simulink model "pet_functional_architecture"  (R2024a)
settings: Solver=FixedStepDiscrete  StartTime=0.0  StopTime=10.0  RelTol=1e-3
undefined symbols (not defined in the file): D1, P
(part 2 of 2)

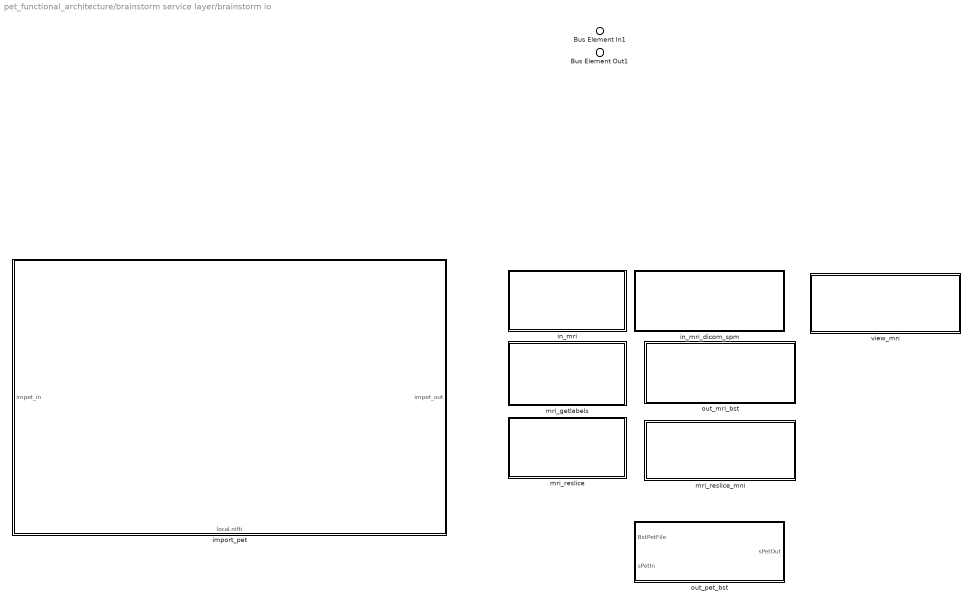
== system pet_functional_architecture/brainstorm service layer/brainstorm io ==
  Bus Element In1 : Inport  AllowServiceAccess=on  PortName=in_(@varargin)
  " out_pet_bst" : Subsystem
      settings: PortSchema="{\"entries\":[{\"content\":{\"headerSize\":26,\"margin\":15,\"minimumSpacing\":25,\"sides\":[{\"content\":{\"connectorIds\":[\"In1\",\"In2\"]},\"type\":\"ConnectorPlacement.EquallySpacedRectSide\",\"uuid\":\"231a4a51-e9d6-4ee1-a9d5-4e29b655c305\"},{\"content\":{\"connectorIds\":[\"Out1\"],\"side\":\"RIGHT\"},\"type\":\"ConnectorPlacement.EquallySpacedRectSide\",\"uuid\":\"e9ceff5f-0784-495f-ae83-524709d043d6\"},{\"content\":{\"side\":\"TOP\"},\"type\":\"ConnectorPlacement.EquallySpacedRectSide\",\"uuid\":\"01c193fb-23d5-46fa-9f50-f56eecaefc77\"}]},\"type\":\"ConnectorPlacement.EquallySpacedConnector\",\"uuid\":\"bc597724-759a-481a-a480-4165a84a707f\"}],\"packageUris\":[\"http://schema.mathworks.com/mf0/Connector/R2020b\"],\"version\":\"1.0\"}"
  import_pet : Subsystem
      settings: PortSchema="{\"entries\":[{\"content\":{\"headerSize\":26,\"margin\":15,\"minimumSpacing\":25,\"sides\":[{\"content\":{\"connectorIds\":[\"In1\"]},\"type\":\"ConnectorPlacement.EquallySpacedRectSide\",\"uuid\":\"e452b68a-48a0-46a4-9e6b-6a7ab63d76ba\"},{\"content\":{\"connectorIds\":[\"Out1\"],\"side\":\"RIGHT\"},\"type\":\"ConnectorPlacement.EquallySpacedRectSide\",\"uuid\":\"bfc23a96-7562-4108-a377-c6d682106293\"},{\"content\":{\"side\":\"TOP\"},\"type\":\"ConnectorPlacement.EquallySpacedRectSide\",\"uuid\":\"898805eb-9365-4e37-9830-3cdbb7191da7\"},{\"content\":{\"connectorIds\":[\"In2\"],\"side\":\"BOTTOM\"},\"type\":\"ConnectorPlacement.EquallySpacedRectSide\",\"uuid\":\"20ed5406-47d9-41fc-b360-c996f9e858c0\"}]},\"type\":\"ConnectorPlacement.EquallySpacedConnector\",\"uuid\":\"9a83eb3e-c81f-4df4-a7ca-e8a116b52f55\"}],\"packageUris\":[\"http://schema.mathworks.com/mf0/Connector/R2020b\"],\"version\":\"1.0\"}"
  in_mri : Subsystem
      settings: PortSchema="{\"entries\":[{\"content\":{\"headerSize\":26,\"margin\":15,\"minimumSpacing\":25,\"sides\":[{\"content\":{},\"type\":\"ConnectorPlacement.EquallySpacedRectSide\",\"uuid\":\"231a4a51-e9d6-4ee1-a9d5-4e29b655c305\"},{\"content\":{\"side\":\"RIGHT\"},\"type\":\"ConnectorPlacement.EquallySpacedRectSide\",\"uuid\":\"e9ceff5f-0784-495f-ae83-524709d043d6\"},{\"content\":{\"side\":\"TOP\"},\"type\":\"ConnectorPlacement.EquallySpacedRectSide\",\"uuid\":\"01c193fb-23d5-46fa-9f50-f56eecaefc77\"}]},\"type\":\"ConnectorPlacement.EquallySpacedConnector\",\"uuid\":\"bc597724-759a-481a-a480-4165a84a707f\"}],\"packageUris\":[\"http://schema.mathworks.com/mf0/Connector/R2020b\"],\"version\":\"1.0\"}"
  in_mri_dicom_spm : Subsystem
      settings: PortSchema="{\"entries\":[{\"content\":{\"headerSize\":26,\"margin\":15,\"minimumSpacing\":25,\"sides\":[{\"content\":{},\"type\":\"ConnectorPlacement.EquallySpacedRectSide\",\"uuid\":\"231a4a51-e9d6-4ee1-a9d5-4e29b655c305\"},{\"content\":{\"side\":\"RIGHT\"},\"type\":\"ConnectorPlacement.EquallySpacedRectSide\",\"uuid\":\"e9ceff5f-0784-495f-ae83-524709d043d6\"},{\"content\":{\"side\":\"TOP\"},\"type\":\"ConnectorPlacement.EquallySpacedRectSide\",\"uuid\":\"01c193fb-23d5-46fa-9f50-f56eecaefc77\"}]},\"type\":\"ConnectorPlacement.EquallySpacedConnector\",\"uuid\":\"bc597724-759a-481a-a480-4165a84a707f\"}],\"packageUris\":[\"http://schema.mathworks.com/mf0/Connector/R2020b\"],\"version\":\"1.0\"}"
  mri_getlabels : Subsystem
      settings: PortSchema="{\"entries\":[{\"content\":{\"headerSize\":26,\"margin\":15,\"minimumSpacing\":25,\"sides\":[{\"content\":{},\"type\":\"ConnectorPlacement.EquallySpacedRectSide\",\"uuid\":\"231a4a51-e9d6-4ee1-a9d5-4e29b655c305\"},{\"content\":{\"side\":\"RIGHT\"},\"type\":\"ConnectorPlacement.EquallySpacedRectSide\",\"uuid\":\"e9ceff5f-0784-495f-ae83-524709d043d6\"},{\"content\":{\"side\":\"TOP\"},\"type\":\"ConnectorPlacement.EquallySpacedRectSide\",\"uuid\":\"01c193fb-23d5-46fa-9f50-f56eecaefc77\"}]},\"type\":\"ConnectorPlacement.EquallySpacedConnector\",\"uuid\":\"bc597724-759a-481a-a480-4165a84a707f\"}],\"packageUris\":[\"http://schema.mathworks.com/mf0/Connector/R2020b\"],\"version\":\"1.0\"}"
  mri_reslice : Subsystem
      settings: PortSchema="{\"entries\":[{\"content\":{\"headerSize\":26,\"margin\":15,\"minimumSpacing\":25,\"sides\":[{\"content\":{},\"type\":\"ConnectorPlacement.EquallySpacedRectSide\",\"uuid\":\"231a4a51-e9d6-4ee1-a9d5-4e29b655c305\"},{\"content\":{\"side\":\"RIGHT\"},\"type\":\"ConnectorPlacement.EquallySpacedRectSide\",\"uuid\":\"e9ceff5f-0784-495f-ae83-524709d043d6\"},{\"content\":{\"side\":\"TOP\"},\"type\":\"ConnectorPlacement.EquallySpacedRectSide\",\"uuid\":\"01c193fb-23d5-46fa-9f50-f56eecaefc77\"}]},\"type\":\"ConnectorPlacement.EquallySpacedConnector\",\"uuid\":\"bc597724-759a-481a-a480-4165a84a707f\"}],\"packageUris\":[\"http://schema.mathworks.com/mf0/Connector/R2020b\"],\"version\":\"1.0\"}"
  mri_reslice_mni : Subsystem
      settings: PortSchema="{\"entries\":[{\"content\":{\"headerSize\":26,\"margin\":15,\"minimumSpacing\":25,\"sides\":[{\"content\":{},\"type\":\"ConnectorPlacement.EquallySpacedRectSide\",\"uuid\":\"231a4a51-e9d6-4ee1-a9d5-4e29b655c305\"},{\"content\":{\"side\":\"RIGHT\"},\"type\":\"ConnectorPlacement.EquallySpacedRectSide\",\"uuid\":\"e9ceff5f-0784-495f-ae83-524709d043d6\"},{\"content\":{\"side\":\"TOP\"},\"type\":\"ConnectorPlacement.EquallySpacedRectSide\",\"uuid\":\"01c193fb-23d5-46fa-9f50-f56eecaefc77\"}]},\"type\":\"ConnectorPlacement.EquallySpacedConnector\",\"uuid\":\"bc597724-759a-481a-a480-4165a84a707f\"}],\"packageUris\":[\"http://schema.mathworks.com/mf0/Connector/R2020b\"],\"version\":\"1.0\"}"
  out_mri_bst : Subsystem
      settings: PortSchema="{\"entries\":[{\"content\":{\"headerSize\":26,\"margin\":15,\"minimumSpacing\":25,\"sides\":[{\"content\":{},\"type\":\"ConnectorPlacement.EquallySpacedRectSide\",\"uuid\":\"231a4a51-e9d6-4ee1-a9d5-4e29b655c305\"},{\"content\":{\"side\":\"RIGHT\"},\"type\":\"ConnectorPlacement.EquallySpacedRectSide\",\"uuid\":\"e9ceff5f-0784-495f-ae83-524709d043d6\"},{\"content\":{\"side\":\"TOP\"},\"type\":\"ConnectorPlacement.EquallySpacedRectSide\",\"uuid\":\"01c193fb-23d5-46fa-9f50-f56eecaefc77\"}]},\"type\":\"ConnectorPlacement.EquallySpacedConnector\",\"uuid\":\"bc597724-759a-481a-a480-4165a84a707f\"}],\"packageUris\":[\"http://schema.mathworks.com/mf0/Connector/R2020b\"],\"version\":\"1.0\"}"
  view_mri : Subsystem
      settings: PortSchema="{\"entries\":[{\"content\":{\"headerSize\":26,\"margin\":15,\"minimumSpacing\":25,\"sides\":[{\"content\":{},\"type\":\"ConnectorPlacement.EquallySpacedRectSide\",\"uuid\":\"231a4a51-e9d6-4ee1-a9d5-4e29b655c305\"},{\"content\":{\"side\":\"RIGHT\"},\"type\":\"ConnectorPlacement.EquallySpacedRectSide\",\"uuid\":\"e9ceff5f-0784-495f-ae83-524709d043d6\"},{\"content\":{\"side\":\"TOP\"},\"type\":\"ConnectorPlacement.EquallySpacedRectSide\",\"uuid\":\"01c193fb-23d5-46fa-9f50-f56eecaefc77\"}]},\"type\":\"ConnectorPlacement.EquallySpacedConnector\",\"uuid\":\"bc597724-759a-481a-a480-4165a84a707f\"}],\"packageUris\":[\"http://schema.mathworks.com/mf0/Connector/R2020b\"],\"version\":\"1.0\"}"
  Bus Element Out1 : Outport  PortName=out_(@varargin)

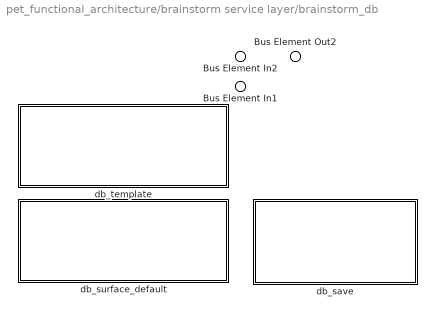
== system pet_functional_architecture/brainstorm service layer/brainstorm_db ==
  Bus Element In1 : Inport  PortName=db_get
  Bus Element In2 : Inport  Port=2  PortName=fcnCall
  db_save : Subsystem
      settings: PortSchema="{\"entries\":[{\"content\":{\"headerSize\":26,\"margin\":15,\"minimumSpacing\":25,\"sides\":[{\"content\":{},\"type\":\"ConnectorPlacement.EquallySpacedRectSide\",\"uuid\":\"231a4a51-e9d6-4ee1-a9d5-4e29b655c305\"},{\"content\":{\"side\":\"RIGHT\"},\"type\":\"ConnectorPlacement.EquallySpacedRectSide\",\"uuid\":\"e9ceff5f-0784-495f-ae83-524709d043d6\"},{\"content\":{\"side\":\"TOP\"},\"type\":\"ConnectorPlacement.EquallySpacedRectSide\",\"uuid\":\"01c193fb-23d5-46fa-9f50-f56eecaefc77\"}]},\"type\":\"ConnectorPlacement.EquallySpacedConnector\",\"uuid\":\"bc597724-759a-481a-a480-4165a84a707f\"}],\"packageUris\":[\"http://schema.mathworks.com/mf0/Connector/R2020b\"],\"version\":\"1.0\"}"
  db_surface_default : Subsystem
      settings: PortSchema="{\"entries\":[{\"content\":{\"headerSize\":26,\"margin\":15,\"minimumSpacing\":25,\"sides\":[{\"content\":{},\"type\":\"ConnectorPlacement.EquallySpacedRectSide\",\"uuid\":\"231a4a51-e9d6-4ee1-a9d5-4e29b655c305\"},{\"content\":{\"side\":\"RIGHT\"},\"type\":\"ConnectorPlacement.EquallySpacedRectSide\",\"uuid\":\"e9ceff5f-0784-495f-ae83-524709d043d6\"},{\"content\":{\"side\":\"TOP\"},\"type\":\"ConnectorPlacement.EquallySpacedRectSide\",\"uuid\":\"01c193fb-23d5-46fa-9f50-f56eecaefc77\"}]},\"type\":\"ConnectorPlacement.EquallySpacedConnector\",\"uuid\":\"bc597724-759a-481a-a480-4165a84a707f\"}],\"packageUris\":[\"http://schema.mathworks.com/mf0/Connector/R2020b\"],\"version\":\"1.0\"}"
  db_template : Subsystem
      settings: PortSchema="{\"entries\":[{\"content\":{\"headerSize\":26,\"margin\":15,\"minimumSpacing\":25,\"sides\":[{\"content\":{},\"type\":\"ConnectorPlacement.EquallySpacedRectSide\",\"uuid\":\"231a4a51-e9d6-4ee1-a9d5-4e29b655c305\"},{\"content\":{\"side\":\"RIGHT\"},\"type\":\"ConnectorPlacement.EquallySpacedRectSide\",\"uuid\":\"e9ceff5f-0784-495f-ae83-524709d043d6\"},{\"content\":{\"side\":\"TOP\"},\"type\":\"ConnectorPlacement.EquallySpacedRectSide\",\"uuid\":\"01c193fb-23d5-46fa-9f50-f56eecaefc77\"}]},\"type\":\"ConnectorPlacement.EquallySpacedConnector\",\"uuid\":\"bc597724-759a-481a-a480-4165a84a707f\"}],\"packageUris\":[\"http://schema.mathworks.com/mf0/Connector/R2020b\"],\"version\":\"1.0\"}"
  Bus Element Out2 : Outport  PortName=db_set

== system pet_functional_architecture/brainstorm tools/ java_getfile ==

== system pet_functional_architecture/brainstorm tools/Anatomy ==
  Bus Element Out2 : Outport  AllowServiceAccess=on  PortName=Surface Recon
  Bus Element Out1 : Outport  Port=2  AllowServiceAccess=on  PortName=BstMriFile

== system pet_functional_architecture/brainstorm tools/bst_colormaps ==

== system pet_functional_architecture/brainstorm tools/bst_fileparts ==

== system pet_functional_architecture/brainstorm tools/bst_flip ==

== system pet_functional_architecture/brainstorm tools/bst_fullfile ==

== system pet_functional_architecture/brainstorm tools/bst_get ==
  Bus Element In2 : Inport  PortName=bst_get(@db)
  Out Bus Element1 : Outport  PortName=io

== system pet_functional_architecture/brainstorm tools/bst_history ==

== system pet_functional_architecture/brainstorm tools/bst_memory ==

== system pet_functional_architecture/brainstorm tools/bst_progress ==

== system pet_functional_architecture/brainstorm tools/bst_set ==
  Bus Element In1 : Inport  PortName=io
  Out Bus Element1 : Outport  PortName=bst_set(@db)

== system pet_functional_architecture/brainstorm tools/db_save ==

== system pet_functional_architecture/brainstorm tools/db_surface_default ==

== system pet_functional_architecture/brainstorm tools/db_template ==

== system pet_functional_architecture/brainstorm tools/file_delete ==

== system pet_functional_architecture/brainstorm tools/file_expand_selection ==

== system pet_functional_architecture/brainstorm tools/file_standardize ==

== system pet_functional_architecture/brainstorm tools/in_mri ==

== system pet_functional_architecture/brainstorm tools/in_mri_dicom_spm ==

== system pet_functional_architecture/brainstorm tools/java_dialog ==

== system pet_functional_architecture/brainstorm tools/mri_getlabels ==

== system pet_functional_architecture/brainstorm tools/mri_reslice ==

== system pet_functional_architecture/brainstorm tools/mri_reslice_mni ==

== system pet_functional_architecture/brainstorm tools/out_mri_bst ==

== system pet_functional_architecture/brainstorm tools/panel_protocols ==

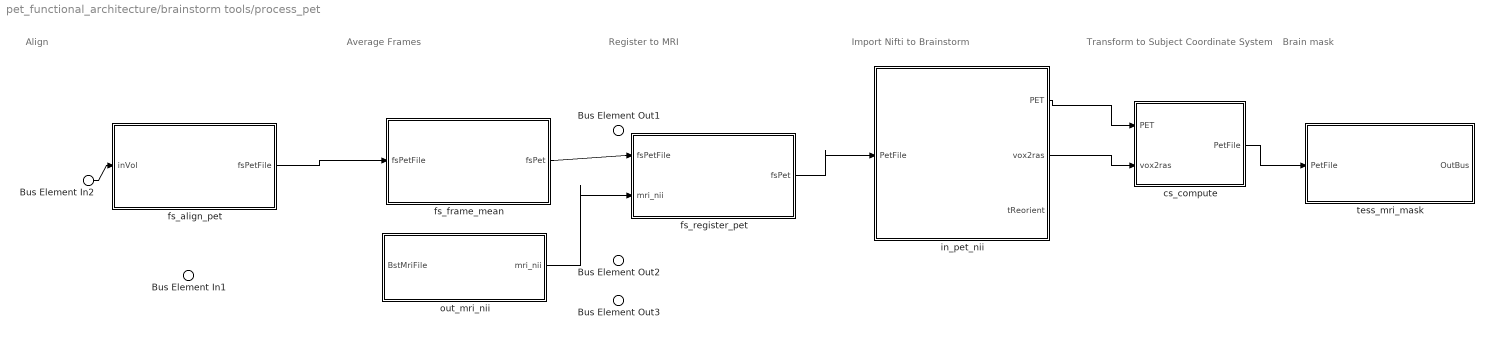
== system pet_functional_architecture/brainstorm tools/process_pet ==
  note: Average Frames
  note: Import Nifti to Brainstorm
  note: Brain mask
  note: Register to MRI
  note: Align
  note: Transform to
      | Subject Coordinate System
  Bus Element In2 : Inport  PortName=PetFile
  Bus Element In1 : Inport  Port=2  AllowServiceAccess=on  PortName=BstMriFile
  cs_compute : Subsystem
      settings: PortSchema="{\"entries\":[{\"content\":{\"headerSize\":26,\"margin\":15,\"minimumSpacing\":25,\"sides\":[{\"content\":{\"connectorIds\":[\"In1\",\"In2\"]},\"type\":\"ConnectorPlacement.EquallySpacedRectSide\",\"uuid\":\"d9face5b-155e-4e83-95c0-d581b737b6e3\"},{\"content\":{\"connectorIds\":[\"Out1\"],\"side\":\"RIGHT\"},\"type\":\"ConnectorPlacement.EquallySpacedRectSide\",\"uuid\":\"f965be1f-1639-4140-b9ea-f5e9efbe4150\"},{\"content\":{\"side\":\"TOP\"},\"type\":\"ConnectorPlacement.EquallySpacedRectSide\",\"uuid\":\"7c9c4b2b-011c-4482-afab-b6e67025a5e2\"}]},\"type\":\"ConnectorPlacement.EquallySpacedConnector\",\"uuid\":\"ec963004-117d-4f22-bb00-71f35201e6e2\"}],\"packageUris\":[\"http://schema.mathworks.com/mf0/Connector/R2020b\"],\"version\":\"1.0\"}"
  fs_align_pet : Subsystem
      settings: PortSchema="{\"entries\":[{\"content\":{\"headerSize\":26,\"margin\":15,\"minimumSpacing\":25,\"sides\":[{\"content\":{\"connectorIds\":[\"In1\"]},\"type\":\"ConnectorPlacement.EquallySpacedRectSide\",\"uuid\":\"d9face5b-155e-4e83-95c0-d581b737b6e3\"},{\"content\":{\"connectorIds\":[\"Out1\"],\"side\":\"RIGHT\"},\"type\":\"ConnectorPlacement.EquallySpacedRectSide\",\"uuid\":\"f965be1f-1639-4140-b9ea-f5e9efbe4150\"},{\"content\":{\"side\":\"TOP\"},\"type\":\"ConnectorPlacement.EquallySpacedRectSide\",\"uuid\":\"7c9c4b2b-011c-4482-afab-b6e67025a5e2\"}]},\"type\":\"ConnectorPlacement.EquallySpacedConnector\",\"uuid\":\"ec963004-117d-4f22-bb00-71f35201e6e2\"}],\"packageUris\":[\"http://schema.mathworks.com/mf0/Connector/R2020b\"],\"version\":\"1.0\"}"
  fs_frame_mean : Subsystem
      settings: PortSchema="{\"entries\":[{\"content\":{\"headerSize\":26,\"margin\":15,\"minimumSpacing\":25,\"sides\":[{\"content\":{\"connectorIds\":[\"In1\"]},\"type\":\"ConnectorPlacement.EquallySpacedRectSide\",\"uuid\":\"d9face5b-155e-4e83-95c0-d581b737b6e3\"},{\"content\":{\"connectorIds\":[\"Out1\"],\"side\":\"RIGHT\"},\"type\":\"ConnectorPlacement.EquallySpacedRectSide\",\"uuid\":\"f965be1f-1639-4140-b9ea-f5e9efbe4150\"},{\"content\":{\"side\":\"TOP\"},\"type\":\"ConnectorPlacement.EquallySpacedRectSide\",\"uuid\":\"7c9c4b2b-011c-4482-afab-b6e67025a5e2\"}]},\"type\":\"ConnectorPlacement.EquallySpacedConnector\",\"uuid\":\"ec963004-117d-4f22-bb00-71f35201e6e2\"}],\"packageUris\":[\"http://schema.mathworks.com/mf0/Connector/R2020b\"],\"version\":\"1.0\"}"
  fs_register_pet : Subsystem
      settings: PortSchema="{\"entries\":[{\"content\":{\"headerSize\":26,\"margin\":15,\"minimumSpacing\":25,\"sides\":[{\"content\":{\"connectorIds\":[\"In1\",\"In2\"]},\"type\":\"ConnectorPlacement.EquallySpacedRectSide\",\"uuid\":\"d9face5b-155e-4e83-95c0-d581b737b6e3\"},{\"content\":{\"connectorIds\":[\"Out1\"],\"side\":\"RIGHT\"},\"type\":\"ConnectorPlacement.EquallySpacedRectSide\",\"uuid\":\"f965be1f-1639-4140-b9ea-f5e9efbe4150\"},{\"content\":{\"side\":\"TOP\"},\"type\":\"ConnectorPlacement.EquallySpacedRectSide\",\"uuid\":\"7c9c4b2b-011c-4482-afab-b6e67025a5e2\"}]},\"type\":\"ConnectorPlacement.EquallySpacedConnector\",\"uuid\":\"ec963004-117d-4f22-bb00-71f35201e6e2\"}],\"packageUris\":[\"http://schema.mathworks.com/mf0/Connector/R2020b\"],\"version\":\"1.0\"}"
  in_pet_nii : Subsystem
      settings: PortSchema="{\"entries\":[{\"content\":{\"headerSize\":26,\"margin\":15,\"minimumSpacing\":25,\"sides\":[{\"content\":{\"connectorIds\":[\"In1\"]},\"type\":\"ConnectorPlacement.EquallySpacedRectSide\",\"uuid\":\"d9face5b-155e-4e83-95c0-d581b737b6e3\"},{\"content\":{\"connectorIds\":[\"Out1\",\"Out2\",\"Out3\"],\"side\":\"RIGHT\"},\"type\":\"ConnectorPlacement.EquallySpacedRectSide\",\"uuid\":\"f965be1f-1639-4140-b9ea-f5e9efbe4150\"},{\"content\":{\"side\":\"TOP\"},\"type\":\"ConnectorPlacement.EquallySpacedRectSide\",\"uuid\":\"7c9c4b2b-011c-4482-afab-b6e67025a5e2\"}]},\"type\":\"ConnectorPlacement.EquallySpacedConnector\",\"uuid\":\"ec963004-117d-4f22-bb00-71f35201e6e2\"}],\"packageUris\":[\"http://schema.mathworks.com/mf0/Connector/R2020b\"],\"version\":\"1.0\"}"
  out_mri_nii : Subsystem
      settings: PortSchema="{\"entries\":[{\"content\":{\"headerSize\":26,\"margin\":15,\"minimumSpacing\":25,\"sides\":[{\"content\":{\"connectorIds\":[\"In1\"]},\"type\":\"ConnectorPlacement.EquallySpacedRectSide\",\"uuid\":\"d9face5b-155e-4e83-95c0-d581b737b6e3\"},{\"content\":{\"connectorIds\":[\"Out1\"],\"side\":\"RIGHT\"},\"type\":\"ConnectorPlacement.EquallySpacedRectSide\",\"uuid\":\"f965be1f-1639-4140-b9ea-f5e9efbe4150\"},{\"content\":{\"side\":\"TOP\"},\"type\":\"ConnectorPlacement.EquallySpacedRectSide\",\"uuid\":\"7c9c4b2b-011c-4482-afab-b6e67025a5e2\"}]},\"type\":\"ConnectorPlacement.EquallySpacedConnector\",\"uuid\":\"ec963004-117d-4f22-bb00-71f35201e6e2\"}],\"packageUris\":[\"http://schema.mathworks.com/mf0/Connector/R2020b\"],\"version\":\"1.0\"}"
  tess_mri_mask : Subsystem
      settings: PortSchema="{\"entries\":[{\"content\":{\"headerSize\":26,\"margin\":15,\"minimumSpacing\":25,\"sides\":[{\"content\":{\"connectorIds\":[\"In1\"]},\"type\":\"ConnectorPlacement.EquallySpacedRectSide\",\"uuid\":\"d9face5b-155e-4e83-95c0-d581b737b6e3\"},{\"content\":{\"connectorIds\":[\"Out1\"],\"side\":\"RIGHT\"},\"type\":\"ConnectorPlacement.EquallySpacedRectSide\",\"uuid\":\"f965be1f-1639-4140-b9ea-f5e9efbe4150\"},{\"content\":{\"side\":\"TOP\"},\"type\":\"ConnectorPlacement.EquallySpacedRectSide\",\"uuid\":\"7c9c4b2b-011c-4482-afab-b6e67025a5e2\"}]},\"type\":\"ConnectorPlacement.EquallySpacedConnector\",\"uuid\":\"ec963004-117d-4f22-bb00-71f35201e6e2\"}],\"packageUris\":[\"http://schema.mathworks.com/mf0/Connector/R2020b\"],\"version\":\"1.0\"}"
  Bus Element Out1 : Outport  PortName=sPet
  Bus Element Out2 : Outport  Port=2  PortName=SUVR Volume
  Bus Element Out3 : Outport  Port=3  PortName=Surface Overlay
  wires:
  Bus Element In2/1 -> fs_align_pet/1(inVol)
  out_mri_nii/1(mri_nii) -> fs_register_pet/2(mri_nii)
  fs_align_pet/1(fsPetFile) -> fs_frame_mean/1(fsPetFile)
  in_pet_nii/2(vox2ras) -> cs_compute/2(vox2ras)
  in_pet_nii/1(PET) -> cs_compute/1(PET)
  fs_frame_mean/1(fsPet) -> fs_register_pet/1(fsPetFile)
  fs_register_pet/1(fsPet) -> in_pet_nii/1(PetFile)
  cs_compute/1(PetFile) -> tess_mri_mask/1(PetFile)

== system pet_functional_architecture/brainstorm tools/view_mri ==

== system pet_functional_architecture/Freesurfer//Brainsuite/Freesurfer/LORIS Data Ingestor ==

== system pet_functional_architecture/Freesurfer//Brainsuite/Freesurfer/Linux ==
  Bus Element In1 : Inport  AllowServiceAccess=on  PortName=Client

== system pet_functional_architecture/Freesurfer//Brainsuite/Freesurfer/Windows ==
  Bus Element In1 : Inport  AllowServiceAccess=on  PortName=Client

== system pet_functional_architecture/Freesurfer//Brainsuite/Freesurfer/gitClone Brainstorm ==
  Bus Element In1 : Inport  AllowServiceAccess=on  PortName=sourceCode

== system pet_functional_architecture/brainstorm service layer/brainstorm core/bst_colormaps ==

== system pet_functional_architecture/brainstorm service layer/brainstorm core/bst_fileparts ==

== system pet_functional_architecture/brainstorm service layer/brainstorm core/bst_flip ==

== system pet_functional_architecture/brainstorm service layer/brainstorm core/bst_fullfile ==

== system pet_functional_architecture/brainstorm service layer/brainstorm core/bst_get ==

== system pet_functional_architecture/brainstorm service layer/brainstorm core/bst_get1 ==
  Bus Element In2 : Inport  PortName=bst_get(@db)
  Out Bus Element1 : Outport  PortName=io

== system pet_functional_architecture/brainstorm service layer/brainstorm core/bst_history ==

== system pet_functional_architecture/brainstorm service layer/brainstorm core/bst_memory ==

== system pet_functional_architecture/brainstorm service layer/brainstorm core/bst_progress ==

== system pet_functional_architecture/brainstorm service layer/brainstorm core/bst_set ==

== system pet_functional_architecture/brainstorm service layer/brainstorm core/bst_set1 ==
  Bus Element In1 : Inport  PortName=io
  Out Bus Element1 : Outport  PortName=bst_set(@db)

== system pet_functional_architecture/brainstorm service layer/brainstorm io/ out_pet_bst ==
  Bus Element In2 : Inport  PortName=BstPetFile
  Bus Element In1 : Inport  Port=2  PortName=sPetIn
  Bus Element Out1 : Outport  PortName=sPetOut

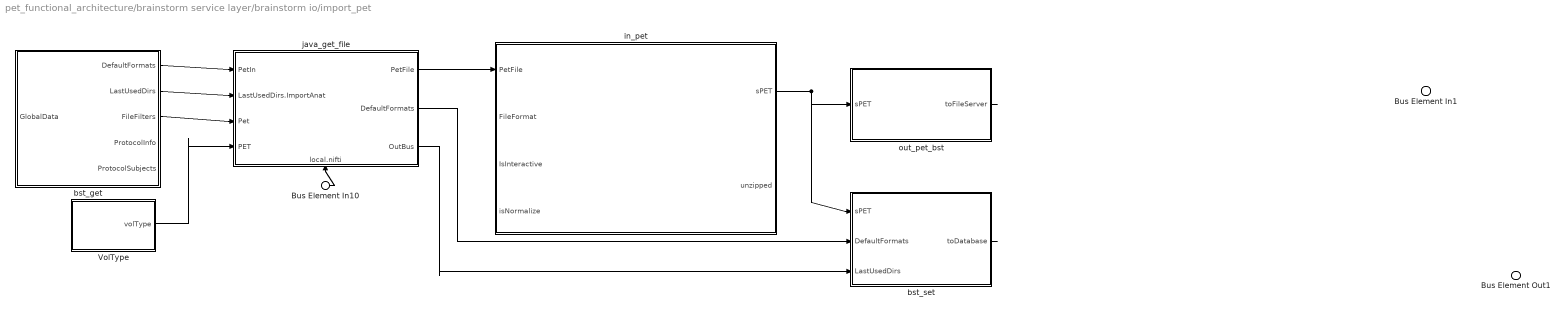
== system pet_functional_architecture/brainstorm service layer/brainstorm io/import_pet ==
  Bus Element In1 : Inport  PortName=impet_in
  Bus Element In10 : Inport  Port=2  AllowServiceAccess=on  PortName=local.nifti
  VolType : Subsystem
      settings: PortSchema="{\"entries\":[{\"content\":{\"headerSize\":26,\"margin\":15,\"minimumSpacing\":25,\"sides\":[{\"content\":{},\"type\":\"ConnectorPlacement.EquallySpacedRectSide\",\"uuid\":\"9dc41937-0423-4f0d-95de-6a11876dea92\"},{\"content\":{\"connectorIds\":[\"Out1\"],\"side\":\"RIGHT\"},\"type\":\"ConnectorPlacement.EquallySpacedRectSide\",\"uuid\":\"a760f902-bb88-44c6-9e15-f93a06bbb22c\"},{\"content\":{\"side\":\"TOP\"},\"type\":\"ConnectorPlacement.EquallySpacedRectSide\",\"uuid\":\"a141426c-a194-4d5c-ba1a-f6f4f49c40a6\"}]},\"type\":\"ConnectorPlacement.EquallySpacedConnector\",\"uuid\":\"ec924d27-401c-47e0-a07a-aece678b254f\"}],\"packageUris\":[\"http://schema.mathworks.com/mf0/Connector/R2020b\"],\"version\":\"1.0\"}"
  bst_get : Subsystem
      settings: PortSchema="{\"entries\":[{\"content\":{\"headerSize\":26,\"margin\":15,\"minimumSpacing\":25,\"sides\":[{\"content\":{\"connectorIds\":[\"In1\"]},\"type\":\"ConnectorPlacement.EquallySpacedRectSide\",\"uuid\":\"e452b68a-48a0-46a4-9e6b-6a7ab63d76ba\"},{\"content\":{\"connectorIds\":[\"Out1\",\"Out2\",\"Out3\",\"Out4\",\"Out5\"],\"side\":\"RIGHT\"},\"type\":\"ConnectorPlacement.EquallySpacedRectSide\",\"uuid\":\"bfc23a96-7562-4108-a377-c6d682106293\"},{\"content\":{\"side\":\"TOP\"},\"type\":\"ConnectorPlacement.EquallySpacedRectSide\",\"uuid\":\"898805eb-9365-4e37-9830-3cdbb7191da7\"}]},\"type\":\"ConnectorPlacement.EquallySpacedConnector\",\"uuid\":\"9a83eb3e-c81f-4df4-a7ca-e8a116b52f55\"}],\"packageUris\":[\"http://schema.mathworks.com/mf0/Connector/R2020b\"],\"version\":\"1.0\"}"
  bst_set : Subsystem
      settings: PortSchema="{\"entries\":[{\"content\":{\"headerSize\":26,\"margin\":15,\"minimumSpacing\":25,\"sides\":[{\"content\":{\"connectorIds\":[\"In1\",\"In2\",\"In3\"]},\"type\":\"ConnectorPlacement.EquallySpacedRectSide\",\"uuid\":\"e452b68a-48a0-46a4-9e6b-6a7ab63d76ba\"},{\"content\":{\"connectorIds\":[\"Out1\"],\"side\":\"RIGHT\"},\"type\":\"ConnectorPlacement.EquallySpacedRectSide\",\"uuid\":\"bfc23a96-7562-4108-a377-c6d682106293\"},{\"content\":{\"side\":\"TOP\"},\"type\":\"ConnectorPlacement.EquallySpacedRectSide\",\"uuid\":\"898805eb-9365-4e37-9830-3cdbb7191da7\"}]},\"type\":\"ConnectorPlacement.EquallySpacedConnector\",\"uuid\":\"9a83eb3e-c81f-4df4-a7ca-e8a116b52f55\"}],\"packageUris\":[\"http://schema.mathworks.com/mf0/Connector/R2020b\"],\"version\":\"1.0\"}"
  in_pet : Subsystem
      settings: PortSchema="{\"entries\":[{\"content\":{\"headerSize\":26,\"margin\":15,\"minimumSpacing\":25,\"sides\":[{\"content\":{\"connectorIds\":[\"In4\",\"In1\",\"In2\",\"In3\"]},\"type\":\"ConnectorPlacement.EquallySpacedRectSide\",\"uuid\":\"e452b68a-48a0-46a4-9e6b-6a7ab63d76ba\"},{\"content\":{\"connectorIds\":[\"Out1\",\"Out2\"],\"side\":\"RIGHT\"},\"type\":\"ConnectorPlacement.EquallySpacedRectSide\",\"uuid\":\"bfc23a96-7562-4108-a377-c6d682106293\"},{\"content\":{\"side\":\"TOP\"},\"type\":\"ConnectorPlacement.EquallySpacedRectSide\",\"uuid\":\"898805eb-9365-4e37-9830-3cdbb7191da7\"}]},\"type\":\"ConnectorPlacement.EquallySpacedConnector\",\"uuid\":\"9a83eb3e-c81f-4df4-a7ca-e8a116b52f55\"}],\"packageUris\":[\"http://schema.mathworks.com/mf0/Connector/R2020b\"],\"version\":\"1.0\"}"
  java_get_file : Subsystem
      settings: PortSchema="{\"entries\":[{\"content\":{\"headerSize\":26,\"margin\":15,\"minimumSpacing\":25,\"sides\":[{\"content\":{\"connectorIds\":[\"In2\",\"In1\",\"In3\",\"In4\"]},\"type\":\"ConnectorPlacement.EquallySpacedRectSide\",\"uuid\":\"d9face5b-155e-4e83-95c0-d581b737b6e3\"},{\"content\":{\"connectorIds\":[\"Out1\",\"Out2\",\"Out3\"],\"side\":\"RIGHT\"},\"type\":\"ConnectorPlacement.EquallySpacedRectSide\",\"uuid\":\"f965be1f-1639-4140-b9ea-f5e9efbe4150\"},{\"content\":{\"side\":\"TOP\"},\"type\":\"ConnectorPlacement.EquallySpacedRectSide\",\"uuid\":\"7c9c4b2b-011c-4482-afab-b6e67025a5e2\"},{\"content\":{\"connectorIds\":[\"In5\"],\"side\":\"BOTTOM\"},\"type\":\"ConnectorPlacement.EquallySpacedRectSide\",\"uuid\":\"d045f323-f36b-4304-ab53-40ed85860a49\"}]},\"type\":\"ConnectorPlacement.EquallySpacedConnector\",\"uuid\":\"ec963004-117d-4f22-bb00-71f35201e6e2\"}],\"packageUris\":[\"http://schema.mathworks.com/mf0/Connector/R2020b\"],\"version\":\"1.0\"}"
  out_pet_bst : Subsystem
      settings: PortSchema="{\"entries\":[{\"content\":{\"headerSize\":26,\"margin\":15,\"minimumSpacing\":25,\"sides\":[{\"content\":{\"connectorIds\":[\"In1\"]},\"type\":\"ConnectorPlacement.EquallySpacedRectSide\",\"uuid\":\"b493315f-c6c8-42ab-8e4d-b8fe240af9dd\"},{\"content\":{\"connectorIds\":[\"Out1\"],\"side\":\"RIGHT\"},\"type\":\"ConnectorPlacement.EquallySpacedRectSide\",\"uuid\":\"94c0e42b-c474-4070-8a16-a26ac22942e6\"},{\"content\":{\"side\":\"TOP\"},\"type\":\"ConnectorPlacement.EquallySpacedRectSide\",\"uuid\":\"f9bc43e9-5c3a-451c-b434-9225c48927cc\"}]},\"type\":\"ConnectorPlacement.EquallySpacedConnector\",\"uuid\":\"067458af-ee7c-44e6-8802-98d558b25815\"}],\"packageUris\":[\"http://schema.mathworks.com/mf0/Connector/R2020b\"],\"version\":\"1.0\"}"
  Bus Element Out1 : Outport  PortName=impet_out
  wires:
  bst_get/3(FileFilters) -> java_get_file/3(Pet)
  bst_get/2(LastUsedDirs) -> java_get_file/1(LastUsedDirs.ImportAnat)
  bst_get/1(DefaultFormats) -> java_get_file/2(PetIn)
  Bus Element In10/1 -> java_get_file/5(local.nifti)
  java_get_file/1(PetFile) -> in_pet/4(PetFile)
  java_get_file/2(DefaultFormats) -> bst_set/2(DefaultFormats)
  java_get_file/3(OutBus) -> bst_set/3(LastUsedDirs)
  VolType/1(volType) -> java_get_file/4(PET)
  in_pet/1(sPET) -> bst_set/1(sPET), out_pet_bst/1(sPET)
  out_pet_bst/1(toFileServer) -> ?
  bst_set/1(toDatabase) -> ?

== system pet_functional_architecture/brainstorm service layer/brainstorm io/in_mri ==

== system pet_functional_architecture/brainstorm service layer/brainstorm io/in_mri_dicom_spm ==

== system pet_functional_architecture/brainstorm service layer/brainstorm io/mri_getlabels ==

== system pet_functional_architecture/brainstorm service layer/brainstorm io/mri_reslice ==

== system pet_functional_architecture/brainstorm service layer/brainstorm io/mri_reslice_mni ==

== system pet_functional_architecture/brainstorm service layer/brainstorm io/out_mri_bst ==

== system pet_functional_architecture/brainstorm service layer/brainstorm io/view_mri ==

== system pet_functional_architecture/brainstorm service layer/brainstorm_db/db_save ==

== system pet_functional_architecture/brainstorm service layer/brainstorm_db/db_surface_default ==

== system pet_functional_architecture/brainstorm service layer/brainstorm_db/db_template ==

== system pet_functional_architecture/brainstorm tools/process_pet/cs_compute ==
  Bus Element In1 : Inport  PortName=PET
  Bus Element In2 : Inport  Port=2  PortName=vox2ras
  Bus Element Out1 : Outport  PortName=PetFile

== system pet_functional_architecture/brainstorm tools/process_pet/fs_align_pet ==
  Bus Element In1 : Inport  PortName=inVol
  Bus Element Out1 : Outport  PortName=fsPetFile

== system pet_functional_architecture/brainstorm tools/process_pet/fs_frame_mean ==
  Bus Element In1 : Inport  PortName=fsPetFile
  Bus Element Out1 : Outport  PortName=fsPet

== system pet_functional_architecture/brainstorm tools/process_pet/fs_register_pet ==
  Bus Element In1 : Inport  PortName=fsPetFile
  Bus Element In2 : Inport  Port=2  PortName=mri_nii
  Bus Element Out1 : Outport  PortName=fsPet

== system pet_functional_architecture/brainstorm tools/process_pet/in_pet_nii ==
  Bus Element In1 : Inport  PortName=PetFile
  Bus Element Out1 : Outport  PortName=PET
  Bus Element Out2 : Outport  Port=2  PortName=vox2ras
  Bus Element Out3 : Outport  Port=3  PortName=tReorient

== system pet_functional_architecture/brainstorm tools/process_pet/out_mri_nii ==
  Bus Element In1 : Inport  AllowServiceAccess=on  PortName=BstMriFile
  Bus Element Out1 : Outport  PortName=mri_nii

== system pet_functional_architecture/brainstorm tools/process_pet/tess_mri_mask ==
  Bus Element In1 : Inport  PortName=PetFile
  Bus Element Out1 : Outport  PortName=OutBus

== system pet_functional_architecture/brainstorm service layer/brainstorm io/import_pet/VolType ==
  Bus Element Out1 : Outport  PortName=volType

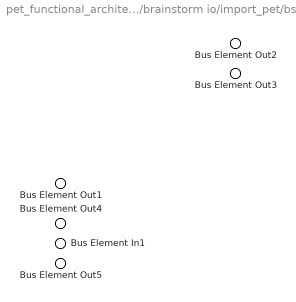
== system pet_functional_architecture/brainstorm service layer/brainstorm io/import_pet/bst_get ==
  Bus Element In1 : Inport  PortName=GlobalData
  Bus Element Out3 : Outport  PortName=DefaultFormats
  Bus Element Out2 : Outport  Port=2  PortName=LastUsedDirs
  Bus Element Out1 : Outport  Port=3  PortName=FileFilters
  Bus Element Out4 : Outport  Port=4  PortName=ProtocolInfo
  Bus Element Out5 : Outport  Port=5  PortName=ProtocolSubjects

== system pet_functional_architecture/brainstorm service layer/brainstorm io/import_pet/bst_set ==
  Bus Element In3 : Inport  PortName=sPET
  Bus Element In1 : Inport  Port=2  PortName=DefaultFormats
  Bus Element In2 : Inport  Port=3  PortName=LastUsedDirs
  Bus Element Out1 : Outport  PortName=toDatabase

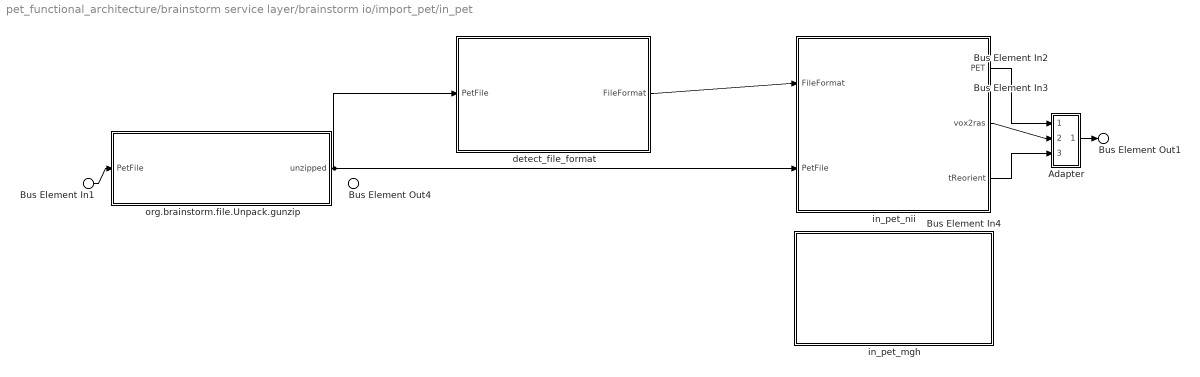
== system pet_functional_architecture/brainstorm service layer/brainstorm io/import_pet/in_pet ==
  Bus Element In2 : Inport  PortName=FileFormat
  Bus Element In3 : Inport  Port=2  PortName=IsInteractive
  Bus Element In4 : Inport  Port=3  PortName=isNormalize
  Bus Element In1 : Inport  Port=4  PortName=PetFile
  Adapter : Subsystem
      settings: PortSchema="{\"entries\":[{\"content\":{\"margin\":10,\"minimumSpacing\":15,\"sides\":[{\"content\":{\"connectorIds\":[\"In1\",\"In2\",\"In3\"]},\"type\":\"ConnectorPlacement.EquallySpacedRectSide\",\"uuid\":\"b493315f-c6c8-42ab-8e4d-b8fe240af9dd\"},{\"content\":{\"connectorIds\":[\"Out1\"],\"side\":\"RIGHT\"},\"type\":\"ConnectorPlacement.EquallySpacedRectSide\",\"uuid\":\"94c0e42b-c474-4070-8a16-a26ac22942e6\"},{\"content\":{\"side\":\"TOP\"},\"type\":\"ConnectorPlacement.EquallySpacedRectSide\",\"uuid\":\"f9bc43e9-5c3a-451c-b434-9225c48927cc\"}]},\"type\":\"ConnectorPlacement.EquallySpacedConnector\",\"uuid\":\"067458af-ee7c-44e6-8802-98d558b25815\"}],\"packageUris\":[\"http://schema.mathworks.com/mf0/Connector/R2020b\"],\"version\":\"1.0\"}"
  detect_file_format : Subsystem
      settings: AttributesFormatString=%<BlockChoice>  PortSchema="{\"entries\":[{\"content\":{\"headerSize\":26,\"margin\":15,\"minimumSpacing\":25,\"sides\":[{\"content\":{\"connectorIds\":[\"In1\"]},\"type\":\"ConnectorPlacement.EquallySpacedRectSide\",\"uuid\":\"e452b68a-48a0-46a4-9e6b-6a7ab63d76ba\"},{\"content\":{\"connectorIds\":[\"Out1\"],\"side\":\"RIGHT\"},\"type\":\"ConnectorPlacement.EquallySpacedRectSide\",\"uuid\":\"bfc23a96-7562-4108-a377-c6d682106293\"},{\"content\":{\"side\":\"TOP\"},\"type\":\"ConnectorPlacement.EquallySpacedRectSide\",\"uuid\":\"898805eb-9365-4e37-9830-3cdbb7191da7\"}]},\"type\":\"ConnectorPlacement.EquallySpacedConnector\",\"uuid\":\"9a83eb3e-c81f-4df4-a7ca-e8a116b52f55\"}],\"packageUris\":[\"http://schema.mathworks.com/mf0/Connector/R2020b\"],\"version\":\"1.0\"}"
  in_pet_mgh : Subsystem  Variant=on  VariantControlMode=label  LabelModeActiveChoice=true
      settings: PortSchema="{\"entries\":[{\"content\":{\"headerSize\":38,\"margin\":15,\"minimumSpacing\":25,\"sides\":[{\"content\":{},\"type\":\"ConnectorPlacement.EquallySpacedRectSide\",\"uuid\":\"b5ae5544-e8bb-4254-ad00-58833e8a7a18\"},{\"content\":{\"side\":\"RIGHT\"},\"type\":\"ConnectorPlacement.EquallySpacedRectSide\",\"uuid\":\"fac4f2c4-a4bc-47a5-a441-dcd98ce2bd10\"},{\"content\":{\"side\":\"TOP\"},\"type\":\"ConnectorPlacement.EquallySpacedRectSide\",\"uuid\":\"59b20440-0331-47da-a238-f55a29059bc4\"}]},\"type\":\"ConnectorPlacement.EquallySpacedConnector\",\"uuid\":\"540bd42e-d22d-4480-8642-7df807d4afe7\"}],\"packageUris\":[\"http://schema.mathworks.com/mf0/Connector/R2020b\"],\"version\":\"1.0\"}"
  in_pet_nii : Subsystem
      settings: PortSchema="{\"entries\":[{\"content\":{\"headerSize\":26,\"margin\":15,\"minimumSpacing\":25,\"sides\":[{\"content\":{\"connectorIds\":[\"In1\",\"In2\"]},\"type\":\"ConnectorPlacement.EquallySpacedRectSide\",\"uuid\":\"9dc41937-0423-4f0d-95de-6a11876dea92\"},{\"content\":{\"connectorIds\":[\"Out1\",\"Out2\",\"Out3\"],\"side\":\"RIGHT\"},\"type\":\"ConnectorPlacement.EquallySpacedRectSide\",\"uuid\":\"a760f902-bb88-44c6-9e15-f93a06bbb22c\"},{\"content\":{\"side\":\"TOP\"},\"type\":\"ConnectorPlacement.EquallySpacedRectSide\",\"uuid\":\"a141426c-a194-4d5c-ba1a-f6f4f49c40a6\"}]},\"type\":\"ConnectorPlacement.EquallySpacedConnector\",\"uuid\":\"ec924d27-401c-47e0-a07a-aece678b254f\"}],\"packageUris\":[\"http://schema.mathworks.com/mf0/Connector/R2020b\"],\"version\":\"1.0\"}"
  org.brainstorm.file.Unpack.gunzip : Subsystem
      settings: PortSchema="{\"entries\":[{\"content\":{\"headerSize\":26,\"margin\":15,\"minimumSpacing\":25,\"sides\":[{\"content\":{\"connectorIds\":[\"In1\"]},\"type\":\"ConnectorPlacement.EquallySpacedRectSide\",\"uuid\":\"e452b68a-48a0-46a4-9e6b-6a7ab63d76ba\"},{\"content\":{\"connectorIds\":[\"Out1\"],\"side\":\"RIGHT\"},\"type\":\"ConnectorPlacement.EquallySpacedRectSide\",\"uuid\":\"bfc23a96-7562-4108-a377-c6d682106293\"},{\"content\":{\"side\":\"TOP\"},\"type\":\"ConnectorPlacement.EquallySpacedRectSide\",\"uuid\":\"898805eb-9365-4e37-9830-3cdbb7191da7\"},{\"content\":{\"side\":\"BOTTOM\"},\"type\":\"ConnectorPlacement.EquallySpacedRectSide\",\"uuid\":\"c4b35227-9c6e-45b4-8456-8559ba2769ae\"}]},\"type\":\"ConnectorPlacement.EquallySpacedConnector\",\"uuid\":\"9a83eb3e-c81f-4df4-a7ca-e8a116b52f55\"}],\"packageUris\":[\"http://schema.mathworks.com/mf0/Connector/R2020b\"],\"version\":\"1.0\"}"
  Bus Element Out1 : Outport  PortName=sPET
  Bus Element Out4 : Outport  Port=2  PortName=unzipped
  wires:
  Bus Element In1/1 -> org.brainstorm.file.Unpack.gunzip/1(PetFile)
  org.brainstorm.file.Unpack.gunzip/1(unzipped) -> detect_file_format/1(PetFile), in_pet_nii/2(PetFile)
  detect_file_format/1(FileFormat) -> in_pet_nii/1(FileFormat)
  in_pet_nii/1(PET) -> Adapter/1(PET)
  in_pet_nii/2(vox2ras) -> Adapter/2(vox2ras)
  in_pet_nii/3(tReorient) -> Adapter/3(tReorient)
  Adapter/1(sPET) -> Bus Element Out1/1

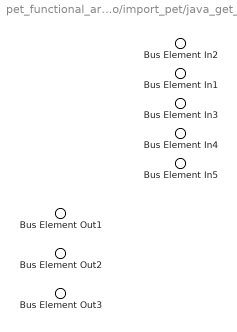
== system pet_functional_architecture/brainstorm service layer/brainstorm io/import_pet/java_get_file ==
  Bus Element In3 : Inport  PortName=LastUsedDirs.ImportAnat
  Bus Element In1 : Inport  Port=2  PortName=PetIn
  Bus Element In4 : Inport  Port=3  PortName=Pet
  Bus Element In5 : Inport  Port=4  PortName=PET
  Bus Element In2 : Inport  Port=5  AllowServiceAccess=on  PortName=local.nifti
  Bus Element Out1 : Outport  PortName=PetFile
  Bus Element Out2 : Outport  Port=2  PortName=DefaultFormats
  Bus Element Out3 : Outport  Port=3  PortName=OutBus

== system pet_functional_architecture/brainstorm service layer/brainstorm io/import_pet/out_pet_bst ==
  Bus Element In1 : Inport  PortName=sPET
  Bus Element Out1 : Outport  PortName=toFileServer

== system pet_functional_architecture/brainstorm service layer/brainstorm io/import_pet/in_pet/Adapter ==
  In Bus Element : Inport  PortName=PET
  Bus Element In2 : Inport  Port=2  PortName=vox2ras
  Bus Element In3 : Inport  Port=3  PortName=tReorient
  Out Bus Element : Outport  PortName=sPET
  wires:
  In Bus Element/1 -> Out Bus Element/1

== system pet_functional_architecture/brainstorm service layer/brainstorm io/import_pet/in_pet/detect_file_format ==
  Bus Element In1 : Inport  PortName=PetFile
  bst_fileparts : Subsystem
      settings: PortSchema="{\"entries\":[{\"content\":{\"headerSize\":26,\"margin\":15,\"minimumSpacing\":25,\"sides\":[{\"content\":{\"connectorIds\":[\"In1\"]},\"type\":\"ConnectorPlacement.EquallySpacedRectSide\",\"uuid\":\"e452b68a-48a0-46a4-9e6b-6a7ab63d76ba\"},{\"content\":{\"connectorIds\":[\"Out1\"],\"side\":\"RIGHT\"},\"type\":\"ConnectorPlacement.EquallySpacedRectSide\",\"uuid\":\"bfc23a96-7562-4108-a377-c6d682106293\"},{\"content\":{\"side\":\"TOP\"},\"type\":\"ConnectorPlacement.EquallySpacedRectSide\",\"uuid\":\"898805eb-9365-4e37-9830-3cdbb7191da7\"}]},\"type\":\"ConnectorPlacement.EquallySpacedConnector\",\"uuid\":\"9a83eb3e-c81f-4df4-a7ca-e8a116b52f55\"}],\"packageUris\":[\"http://schema.mathworks.com/mf0/Connector/R2020b\"],\"version\":\"1.0\"}"
  Bus Element Out1 : Outport  PortName=FileFormat
  wires:
  Bus Element In1/1 -> bst_fileparts/1(PetFile)
  bst_fileparts/1(fExt) -> Bus Element Out1/1

== system pet_functional_architecture/brainstorm service layer/brainstorm io/import_pet/in_pet/in_pet_mgh ==
  in_pet_bst : Subsystem  VariantControl=false
      settings: PortSchema="{\"entries\":[{\"content\":{\"headerSize\":26,\"margin\":15,\"minimumSpacing\":25,\"sides\":[{\"content\":{},\"type\":\"ConnectorPlacement.EquallySpacedRectSide\",\"uuid\":\"72abe335-e3fb-41dd-b80c-12077d308238\"},{\"content\":{\"side\":\"RIGHT\"},\"type\":\"ConnectorPlacement.EquallySpacedRectSide\",\"uuid\":\"ae31e00a-5428-4492-b9cf-7f4d180b4032\"},{\"content\":{\"side\":\"TOP\"},\"type\":\"ConnectorPlacement.EquallySpacedRectSide\",\"uuid\":\"1347eab1-52cf-472f-92d5-2cceb7c753dd\"}]},\"type\":\"ConnectorPlacement.EquallySpacedConnector\",\"uuid\":\"996eae90-ea0d-4e0d-ad72-246c3f6a3cae\"}],\"packageUris\":[\"http://schema.mathworks.com/mf0/Connector/R2020b\"],\"version\":\"1.0\"}"
  in_pet_dicom : Subsystem  VariantControl=Component
      settings: PortSchema="{\"entries\":[{\"content\":{\"headerSize\":26,\"margin\":15,\"minimumSpacing\":25,\"sides\":[{\"content\":{},\"type\":\"ConnectorPlacement.EquallySpacedRectSide\",\"uuid\":\"9dc41937-0423-4f0d-95de-6a11876dea92\"},{\"content\":{\"side\":\"RIGHT\"},\"type\":\"ConnectorPlacement.EquallySpacedRectSide\",\"uuid\":\"a760f902-bb88-44c6-9e15-f93a06bbb22c\"},{\"content\":{\"side\":\"TOP\"},\"type\":\"ConnectorPlacement.EquallySpacedRectSide\",\"uuid\":\"a141426c-a194-4d5c-ba1a-f6f4f49c40a6\"}]},\"type\":\"ConnectorPlacement.EquallySpacedConnector\",\"uuid\":\"ec924d27-401c-47e0-a07a-aece678b254f\"}],\"packageUris\":[\"http://schema.mathworks.com/mf0/Connector/R2020b\"],\"version\":\"1.0\"}"
  in_pet_mgh : Subsystem  VariantControl=true
      settings: PortSchema="{\"entries\":[{\"content\":{\"headerSize\":26,\"margin\":15,\"minimumSpacing\":25,\"sides\":[{\"content\":{},\"type\":\"ConnectorPlacement.EquallySpacedRectSide\",\"uuid\":\"72abe335-e3fb-41dd-b80c-12077d308238\"},{\"content\":{\"side\":\"RIGHT\"},\"type\":\"ConnectorPlacement.EquallySpacedRectSide\",\"uuid\":\"ae31e00a-5428-4492-b9cf-7f4d180b4032\"},{\"content\":{\"side\":\"TOP\"},\"type\":\"ConnectorPlacement.EquallySpacedRectSide\",\"uuid\":\"1347eab1-52cf-472f-92d5-2cceb7c753dd\"}]},\"type\":\"ConnectorPlacement.EquallySpacedConnector\",\"uuid\":\"996eae90-ea0d-4e0d-ad72-246c3f6a3cae\"}],\"packageUris\":[\"http://schema.mathworks.com/mf0/Connector/R2020b\"],\"version\":\"1.0\"}"

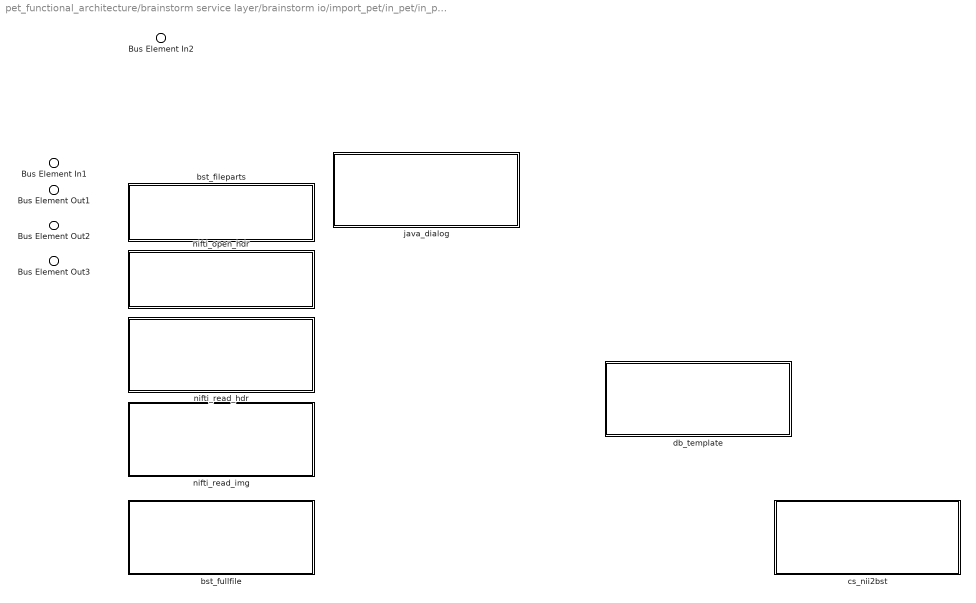
== system pet_functional_architecture/brainstorm service layer/brainstorm io/import_pet/in_pet/in_pet_nii ==
  Bus Element In2 : Inport  PortName=FileFormat
  Bus Element In1 : Inport  Port=2  PortName=PetFile
  bst_fileparts : Subsystem
      settings: PortSchema="{\"entries\":[{\"content\":{\"headerSize\":26,\"margin\":15,\"minimumSpacing\":25,\"sides\":[{\"content\":{},\"type\":\"ConnectorPlacement.EquallySpacedRectSide\",\"uuid\":\"9dc41937-0423-4f0d-95de-6a11876dea92\"},{\"content\":{\"side\":\"RIGHT\"},\"type\":\"ConnectorPlacement.EquallySpacedRectSide\",\"uuid\":\"a760f902-bb88-44c6-9e15-f93a06bbb22c\"},{\"content\":{\"side\":\"TOP\"},\"type\":\"ConnectorPlacement.EquallySpacedRectSide\",\"uuid\":\"a141426c-a194-4d5c-ba1a-f6f4f49c40a6\"}]},\"type\":\"ConnectorPlacement.EquallySpacedConnector\",\"uuid\":\"ec924d27-401c-47e0-a07a-aece678b254f\"}],\"packageUris\":[\"http://schema.mathworks.com/mf0/Connector/R2020b\"],\"version\":\"1.0\"}"
  bst_fullfile : Subsystem
      settings: PortSchema="{\"entries\":[{\"content\":{\"headerSize\":26,\"margin\":15,\"minimumSpacing\":25,\"sides\":[{\"content\":{},\"type\":\"ConnectorPlacement.EquallySpacedRectSide\",\"uuid\":\"9dc41937-0423-4f0d-95de-6a11876dea92\"},{\"content\":{\"side\":\"RIGHT\"},\"type\":\"ConnectorPlacement.EquallySpacedRectSide\",\"uuid\":\"a760f902-bb88-44c6-9e15-f93a06bbb22c\"},{\"content\":{\"side\":\"TOP\"},\"type\":\"ConnectorPlacement.EquallySpacedRectSide\",\"uuid\":\"a141426c-a194-4d5c-ba1a-f6f4f49c40a6\"}]},\"type\":\"ConnectorPlacement.EquallySpacedConnector\",\"uuid\":\"ec924d27-401c-47e0-a07a-aece678b254f\"}],\"packageUris\":[\"http://schema.mathworks.com/mf0/Connector/R2020b\"],\"version\":\"1.0\"}"
  cs_nii2bst : Subsystem
      settings: PortSchema="{\"entries\":[{\"content\":{\"headerSize\":26,\"margin\":15,\"minimumSpacing\":25,\"sides\":[{\"content\":{},\"type\":\"ConnectorPlacement.EquallySpacedRectSide\",\"uuid\":\"9dc41937-0423-4f0d-95de-6a11876dea92\"},{\"content\":{\"side\":\"RIGHT\"},\"type\":\"ConnectorPlacement.EquallySpacedRectSide\",\"uuid\":\"a760f902-bb88-44c6-9e15-f93a06bbb22c\"},{\"content\":{\"side\":\"TOP\"},\"type\":\"ConnectorPlacement.EquallySpacedRectSide\",\"uuid\":\"a141426c-a194-4d5c-ba1a-f6f4f49c40a6\"}]},\"type\":\"ConnectorPlacement.EquallySpacedConnector\",\"uuid\":\"ec924d27-401c-47e0-a07a-aece678b254f\"}],\"packageUris\":[\"http://schema.mathworks.com/mf0/Connector/R2020b\"],\"version\":\"1.0\"}"
  db_template : Subsystem
      settings: PortSchema="{\"entries\":[{\"content\":{\"headerSize\":26,\"margin\":15,\"minimumSpacing\":25,\"sides\":[{\"content\":{},\"type\":\"ConnectorPlacement.EquallySpacedRectSide\",\"uuid\":\"9dc41937-0423-4f0d-95de-6a11876dea92\"},{\"content\":{\"side\":\"RIGHT\"},\"type\":\"ConnectorPlacement.EquallySpacedRectSide\",\"uuid\":\"a760f902-bb88-44c6-9e15-f93a06bbb22c\"},{\"content\":{\"side\":\"TOP\"},\"type\":\"ConnectorPlacement.EquallySpacedRectSide\",\"uuid\":\"a141426c-a194-4d5c-ba1a-f6f4f49c40a6\"}]},\"type\":\"ConnectorPlacement.EquallySpacedConnector\",\"uuid\":\"ec924d27-401c-47e0-a07a-aece678b254f\"}],\"packageUris\":[\"http://schema.mathworks.com/mf0/Connector/R2020b\"],\"version\":\"1.0\"}"
  java_dialog : Subsystem
      settings: PortSchema="{\"entries\":[{\"content\":{\"headerSize\":26,\"margin\":15,\"minimumSpacing\":25,\"sides\":[{\"content\":{},\"type\":\"ConnectorPlacement.EquallySpacedRectSide\",\"uuid\":\"9dc41937-0423-4f0d-95de-6a11876dea92\"},{\"content\":{\"side\":\"RIGHT\"},\"type\":\"ConnectorPlacement.EquallySpacedRectSide\",\"uuid\":\"a760f902-bb88-44c6-9e15-f93a06bbb22c\"},{\"content\":{\"side\":\"TOP\"},\"type\":\"ConnectorPlacement.EquallySpacedRectSide\",\"uuid\":\"a141426c-a194-4d5c-ba1a-f6f4f49c40a6\"}]},\"type\":\"ConnectorPlacement.EquallySpacedConnector\",\"uuid\":\"ec924d27-401c-47e0-a07a-aece678b254f\"}],\"packageUris\":[\"http://schema.mathworks.com/mf0/Connector/R2020b\"],\"version\":\"1.0\"}"
  nifti_open_hdr : Subsystem
      settings: PortSchema="{\"entries\":[{\"content\":{\"headerSize\":26,\"margin\":15,\"minimumSpacing\":25,\"sides\":[{\"content\":{},\"type\":\"ConnectorPlacement.EquallySpacedRectSide\",\"uuid\":\"9dc41937-0423-4f0d-95de-6a11876dea92\"},{\"content\":{\"side\":\"RIGHT\"},\"type\":\"ConnectorPlacement.EquallySpacedRectSide\",\"uuid\":\"a760f902-bb88-44c6-9e15-f93a06bbb22c\"},{\"content\":{\"side\":\"TOP\"},\"type\":\"ConnectorPlacement.EquallySpacedRectSide\",\"uuid\":\"a141426c-a194-4d5c-ba1a-f6f4f49c40a6\"}]},\"type\":\"ConnectorPlacement.EquallySpacedConnector\",\"uuid\":\"ec924d27-401c-47e0-a07a-aece678b254f\"}],\"packageUris\":[\"http://schema.mathworks.com/mf0/Connector/R2020b\"],\"version\":\"1.0\"}"
  nifti_read_hdr : Subsystem
      settings: PortSchema="{\"entries\":[{\"content\":{\"headerSize\":26,\"margin\":15,\"minimumSpacing\":25,\"sides\":[{\"content\":{},\"type\":\"ConnectorPlacement.EquallySpacedRectSide\",\"uuid\":\"9dc41937-0423-4f0d-95de-6a11876dea92\"},{\"content\":{\"side\":\"RIGHT\"},\"type\":\"ConnectorPlacement.EquallySpacedRectSide\",\"uuid\":\"a760f902-bb88-44c6-9e15-f93a06bbb22c\"},{\"content\":{\"side\":\"TOP\"},\"type\":\"ConnectorPlacement.EquallySpacedRectSide\",\"uuid\":\"a141426c-a194-4d5c-ba1a-f6f4f49c40a6\"}]},\"type\":\"ConnectorPlacement.EquallySpacedConnector\",\"uuid\":\"ec924d27-401c-47e0-a07a-aece678b254f\"}],\"packageUris\":[\"http://schema.mathworks.com/mf0/Connector/R2020b\"],\"version\":\"1.0\"}"
  nifti_read_img : Subsystem
      settings: PortSchema="{\"entries\":[{\"content\":{\"headerSize\":26,\"margin\":15,\"minimumSpacing\":25,\"sides\":[{\"content\":{},\"type\":\"ConnectorPlacement.EquallySpacedRectSide\",\"uuid\":\"9dc41937-0423-4f0d-95de-6a11876dea92\"},{\"content\":{\"side\":\"RIGHT\"},\"type\":\"ConnectorPlacement.EquallySpacedRectSide\",\"uuid\":\"a760f902-bb88-44c6-9e15-f93a06bbb22c\"},{\"content\":{\"side\":\"TOP\"},\"type\":\"ConnectorPlacement.EquallySpacedRectSide\",\"uuid\":\"a141426c-a194-4d5c-ba1a-f6f4f49c40a6\"}]},\"type\":\"ConnectorPlacement.EquallySpacedConnector\",\"uuid\":\"ec924d27-401c-47e0-a07a-aece678b254f\"}],\"packageUris\":[\"http://schema.mathworks.com/mf0/Connector/R2020b\"],\"version\":\"1.0\"}"
  Bus Element Out1 : Outport  PortName=PET
  Bus Element Out2 : Outport  Port=2  PortName=vox2ras
  Bus Element Out3 : Outport  Port=3  PortName=tReorient

== system pet_functional_architecture/brainstorm service layer/brainstorm io/import_pet/in_pet/org.brainstorm.file.Unpack.gunzip ==
  Bus Element In1 : Inport  PortName=PetFile
  Bus Element Out1 : Outport  PortName=unzipped

== system pet_functional_architecture/brainstorm service layer/brainstorm io/import_pet/in_pet/detect_file_format/bst_fileparts ==
  Bus Element In1 : Inport  PortName=PetFile
  Bus Element Out1 : Outport  PortName=fExt

== system pet_functional_architecture/brainstorm service layer/brainstorm io/import_pet/in_pet/in_pet_mgh/in_pet_bst ==

== system pet_functional_architecture/brainstorm service layer/brainstorm io/import_pet/in_pet/in_pet_mgh/in_pet_dicom ==

== system pet_functional_architecture/brainstorm service layer/brainstorm io/import_pet/in_pet/in_pet_mgh/in_pet_mgh ==

== system pet_functional_architecture/brainstorm service layer/brainstorm io/import_pet/in_pet/in_pet_nii/bst_fileparts ==

== system pet_functional_architecture/brainstorm service layer/brainstorm io/import_pet/in_pet/in_pet_nii/bst_fullfile ==

== system pet_functional_architecture/brainstorm service layer/brainstorm io/import_pet/in_pet/in_pet_nii/cs_nii2bst ==

== system pet_functional_architecture/brainstorm service layer/brainstorm io/import_pet/in_pet/in_pet_nii/db_template ==

== system pet_functional_architecture/brainstorm service layer/brainstorm io/import_pet/in_pet/in_pet_nii/java_dialog ==

== system pet_functional_architecture/brainstorm service layer/brainstorm io/import_pet/in_pet/in_pet_nii/nifti_open_hdr ==

== system pet_functional_architecture/brainstorm service layer/brainstorm io/import_pet/in_pet/in_pet_nii/nifti_read_hdr ==

== system pet_functional_architecture/brainstorm service layer/brainstorm io/import_pet/in_pet/in_pet_nii/nifti_read_img ==
